simulink model "Initalisation_block"  (R2019b)
settings: Solver=ode3  StartTime=0.0  StopTime=0.01  FixedStep=0.000080  RelTol=1e-3  EnableMultiTasking=on
settings Model: Creator=cary  LastModifiedBy=adshetgaonkar
settings DataIOCC: LimitDataPoints=on  SaveFormat=Array  SignalLoggingSaveFormat=ModelDataLogs  SaveOutput=off  SignalLogging=off  DSMLogging=off  SaveTime=off  ReturnWorkspaceOutputs=off
settings OptimizationCC: ExpressionDepthLimit=2147483647  LifeSpan=1  EfficientTunableParamExpr=on
settings DebuggingCC: UnderspecifiedInitializationDetection=Classic  MergeDetectMultiDrivingBlocksExec=none  SolverPrmCheckMsg=warning  FcnCallInpInsideContextMsg=warning  StateNameClashWarn=warning  SFUnexpectedBacktrackingDiag=warning  SFNoUnconditionalDefaultTransitionDiag=warning  SFExecutionAtInitializationDiag=none  ArithmeticOperatorsInVariantConditions=warning
settings HardwareCC: ProdBitPerPointer=32  ProdBitPerSizeT=32  ProdBitPerPtrDiffT=32  ProdLargestAtomicFloat=None  ProdIntDivRoundTo=Undefined  ProdEndianess=Unspecified  ProdWordSize=32  ProdHWDeviceType=32-bit Generic
settings ModelReferenceCC: PropagateSignalLabelsOutOfModel=off
settings SFSimCC: SimUseLocalCustomCode=off  MATLABDynamicMemAlloc=off  CustomCodeUndefinedFunction=UseInterfaceOnly
settings RTWCC: SystemTargetFile=ert.tlc  TemplateMakefile=ert_default_tmf  RTWUseLocalCustomCode=off
settings CodeAppCC: IgnoreCustomStorageClasses=off  CustomSymbolStrType=$N$R$M  StateflowObjectComments=on  InternalIdentifier=Classic
settings ERTTargetCC: MultiwordLength=2048  GenerateSampleERTMain=on  IncludeMdlTerminateFcn=off  SupportComplex=off  SupportContinuousTime=on  SupportVariableSizeSignals=on  ERTCustomFileTemplate=example_file_process.tlc  ConvertIfToSwitch=off  SuppressUnreachableDefaultCases=off
settings ConfigComp: CovMetricSettings=dw  CovHtmlReporting=on  CovSaveCumulativeToWorkspaceVar=on  CovSaveSingleToWorkspaceVar=on  CovExternalEMLEnable=off

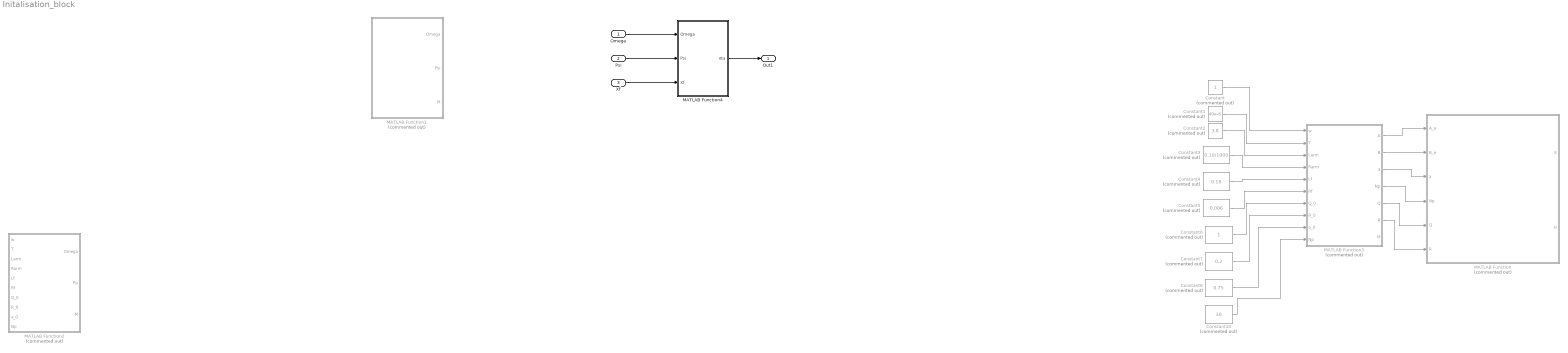
== system Initalisation_block ==
  Omega : Inport  PortDimensions=[20 20]
  Psi : Inport  Port=2  PortDimensions=[20 10]
  Xf : Inport  Port=3  PortDimensions=[10 1]
  Constant : Constant  Commented=on
  Constant1 : Constant  Commented=on  Value=40e-6
  Constant10 : Constant  Commented=on  Value=30
  Constant2 : Constant  Commented=on  Value=3.8
  Constant3 : Constant  Commented=on  Value=0.10/1000
  Constant4 : Constant  Commented=on  Value=0.18
  Constant5 : Constant  Commented=on  Value=0.006
  Constant6 : Constant  Commented=on
  Constant7 : Constant  Commented=on  Value=0.2
  Constant8 : Constant  Commented=on  Value=0.75
  MATLAB Function : MATLAB Function  Commented=on  TreatAsAtomicUnit=on
  MATLAB Function1 : MATLAB Function  Commented=on  TreatAsAtomicUnit=on
  MATLAB Function2 : MATLAB Function  Commented=on  TreatAsAtomicUnit=on
  MATLAB Function3 : MATLAB Function  Commented=on  TreatAsAtomicUnit=on
  MATLAB Function4 : MATLAB Function  TreatAsAtomicUnit=on
  Out1 : Outport  SignalName=eta
  wires:
  MATLAB Function3/1(A) -> MATLAB Function/1(A_e)
  MATLAB Function3/2(B) -> MATLAB Function/2(B_e)
  MATLAB Function3/3(a) -> MATLAB Function/3(a)
  MATLAB Function3/4(Np) -> MATLAB Function/4(Np)
  MATLAB Function3/5(Q) -> MATLAB Function/5(Q)
  MATLAB Function3/6(R) -> MATLAB Function/6(R)
  Constant1/1 -> MATLAB Function3/2(T)
  Constant/1 -> MATLAB Function3/1(w)
  Constant2/1 -> MATLAB Function3/3(Larm)
  Constant3/1 -> MATLAB Function3/4(Rarm)
  Constant4/1 -> MATLAB Function3/5(Lf)
  Constant5/1 -> MATLAB Function3/6(Rf)
  Constant6/1 -> MATLAB Function3/7(Q_0)
  Constant7/1 -> MATLAB Function3/8(R_0)
  Constant8/1 -> MATLAB Function3/9(a_0)
  Constant10/1 -> MATLAB Function3/10("Np ")
  Omega/1 -> MATLAB Function4/1(Omega)
  Psi/1 -> MATLAB Function4/2(Psi)
  Xf/1 -> MATLAB Function4/3(Xf)
  MATLAB Function4/1(eta) -> Out1/1

== matlab function Initalisation_block/MATLAB Function1 ==
  data: Omega output; Psi output; M output [1..100]
function [Omega,Psi,M] = fcn()
D = []; 
D = coder.load('initial_qudratic_papervx.mat');

Omega = D.Omega; 

Psi = D.Psi;

M = D.M;
end

== matlab function Initalisation_block/MATLAB Function2 ==
  data: Omega output; Psi output; w input size=1; M output [1..100]; T input size=1; Larm input size=1; Rarm input size=1; Lf input size=1; Rf input size=1; Q_0 input size=1; R_0 input size=1; a_0 input size=1; Np input size=1
function [Omega,Psi,M] = fcn(w,T,Larm,Rarm,Lf,Rf,Q_0,R_0,a_0,Np)
%w = 1; 
%T =0.2e-3; 
% T = 30e-6; %%%%% very important for simple circuit with 1e-6 it works
% Larm =  1.1;
% Rarm = 0.10/1000

%T = 40e-6; %%%%% very important for simple circuit with 1e-6 it works
%Larm = 3.8;  %%1.5 %%3.8
%Rarm = 0.10/1000; %%%0.10/1000;

%Lf = 0.18;
%Rf = 0.006; %Rf = 0.006;
%%
R_ac_eq = Rf + Rarm/2;  
L_ac_eq = Lf + Larm/2; 
R_dc_eq = 2*Rarm; 
L_dc_eq = 2*Larm;

A_ac = [-Rarm/Larm 2*w 0 0 0; -2*w -Rarm/Larm 0 0 0; 0 0 -Rarm/Larm 0 0; ...
        0 0 0  -R_ac_eq/L_ac_eq -w; 0 0 0 w -R_ac_eq/L_ac_eq ]; 
B_ac = [-1/Larm 0 0 0 0; 0 -1/Larm 0 0 0; 0 0 -1/Larm 0 0;
         0 0 0 1/L_ac_eq 0 ; 0 0 0 0 1/L_ac_eq ];

[Na_r,Na_c] = size(A_ac); 
[Nb_r,Nb_c] = size(B_ac);
C_ac = eye(Na_r,Nb_r); 
D_ac = zeros(Na_r,Nb_c);

F = expm(A_ac*T); 
G = A_ac\((expm(A_ac*T)- eye([Na_r,Na_c]))*B_ac);

Ap_ac = F; 
Bp_ac = G; 
Cp_ac = C_ac; 
%%%%%%%%%%%%%%%%%%%%%%%%%%%%%%%
[m1,n1]=size(Cp_ac);
[n1,n_in]=size(Bp_ac);
A=eye(n1+m1,n1+m1);
A(1:n1,1:n1)=Ap_ac;
A(n1+1:n1+m1,1:n1)=Cp_ac*Ap_ac;
B=zeros(n1+m1,n_in);
B(1:n1,:)=Bp_ac;
B(n1+1:n1+m1,:)=Cp_ac*Bp_ac;
C=zeros(m1,n1+m1);
C(:,n1+1:n1+m1)=eye(m1,m1);

%%
%Q_0 = 1;
%R_0 = 0.2;
%a_0 =0.75;
Q= Q_0*C'*C;
%Q=[0 0 0 0; 0 0 0 0; 0 0 100 0;  0 0 0 100]; %% check for effect of Q 
R=R_0*eye(n_in,n_in);
%R=0.9*eye(n_in,n_in)
a=a_0*ones (n_in,1);
N= 4*ones (n_in,1); %you can increase N
%Np=45;
%Np=30;
[Omega,Psi]= dmpc(A,B,a,N,Np,Q,R); 
%%%
%%
xm=zeros(n1,1);
N_sim = 300;
y=zeros(m1,1);
u=zeros(n_in,1);
xm=zeros(n1,1);
%%%%%%%%%%refrence %%%%%%%

r = zeros(m1,1);
Xf=[xm;(y-r)];
u_min= -0.3*ones (n_in,1);
u_max= 0.3*ones (n_in,1);
deltau_min = -10*ones (n_in,1);
deltau_max = 10*ones (n_in,1);
up=zeros(n_in,1);
%[M,Lzerot]=Mdu(a,N,n_in,1); %% for contrain on the rate
%[M0]= Mu(a,N,n_in,2); %%% for contrain on the amplitude 
%% contrain on both rate and amplitude
[M1,Lzerot]=Mdu(a,N,n_in,1);
M0=Mu(a,N,n_in,1);
M=[M0;-M0;M1;-M1];

end

== matlab function Initalisation_block/MATLAB Function ==
  data: A_e input; E output; B_e input; a input; Np input; Q input; R input; H output
 function [E,H] =fcn(A_e,B_e,a,Np,Q,R)
%A_e;B_e define the extended state-space model when
% integrator is used
%they can also be other forms of state-space models
% a contains the Laguerre pole locations for each input
%N the number of terms for each input
%Np prediction horizon
%Q weight on the state variables
%R weight on the input variables assumed to be diagonal.
% The cost function is J= eta ^T E eta +2 eta ^T H x(k_i)
[n,n_in]=size(B_e);
N= 4*ones (n_in,1);
N_pa=sum(N); %the dimension of eta
E=zeros(N_pa,N_pa);
H=zeros(N_pa,n);
R_para=zeros(N_pa,N_pa);
n0=1;
ne=N(1);
for i=1:n_in-1
R_para(n0:ne,n0:ne)= R(i,i)*eye(N(i),N(i));
n0=n0+N(i);
ne=ne+N(i+1);
end
R_para(n0:N_pa,n0:N_pa)=R(n_in,n_in)*eye(N(n_in),N(n_in));
S_in=zeros(n,N_pa);
[Al,L0]=lagd(a(1),N(1));
S_in(:,1:N(1))=B_e(:,1)*L0';
In_s=1;
for jj=2:n_in
[Al,L0]=lagd(a(jj),N(jj));
In_s=N(jj-1)+In_s;
In_e=In_s+N(jj)-1;
S_in(:,In_s:In_e)=B_e(:,jj)*L0';
end
S_sum = S_in;
phi=S_in;
E=(phi)'*Q*(phi);
H=phi'*Q*A_e;
for i=2:Np
Eae=A_e^i;
%calculate the finite sum S for each input
%%%%%%%%%%%%%%%%%%%%%%%%%%%%%%%%%%%%%%%
%For each sample i
%%%%%%%%%%%%calculate input number 1
%specify the L0 and state matrix Al
%associated with the first input
[Al,L0]=lagd(a(1),N(1));
% Laguerre function associated with input number 1
S_sum(:,1:N(1))=A_e*S_sum(:,1:N(1))+ S_in(:,1:N(1))*(Al^(i-1))';
%%move on to input number 2 and so on
In_s=1;
for kk=2:n_in
[Al,L0]=lagd(a(kk),N(kk));
In_s=N(kk-1)+In_s;
In_e=In_s+N(kk)-1;
S_sum(:,In_s:In_e)=A_e*S_sum(:,In_s:In_e)+ S_in(:,In_s:In_e)*(Al^(i-1))';
end
phi=S_sum;
E=E+phi'*Q*phi;
H=H+phi'*Q*Eae;
end
E=E+R_para;

== matlab function Initalisation_block/MATLAB Function3 ==
  data: w input; A output; T input; Larm input; Rarm input; Lf input; Rf input; Q_0 input; R_0 input; a_0 input; B output; a output; Np output; Q output; R output; Np input; M output
function [A,B,a,Np,Q,R,M] = fcn(w,T,Larm,Rarm,Lf,Rf,Q_0,R_0,a_0,Np)
%w = 1; 
%T =0.2e-3; 
% T = 30e-6; %%%%% very important for simple circuit with 1e-6 it works
% Larm =  1.1;
% Rarm = 0.10/1000

%T = 40e-6; %%%%% very important for simple circuit with 1e-6 it works
%Larm = 3.8;  %%1.5 %%3.8
%Rarm = 0.10/1000; %%%0.10/1000;

%Lf = 0.18;
%Rf = 0.006; %Rf = 0.006;
%%
R_ac_eq = Rf + Rarm/2;  
L_ac_eq = Lf + Larm/2; 
R_dc_eq = 2*Rarm; 
L_dc_eq = 2*Larm;

A_ac = [-Rarm/Larm 2*w 0 0 0; -2*w -Rarm/Larm 0 0 0; 0 0 -Rarm/Larm 0 0; ...
        0 0 0  -R_ac_eq/L_ac_eq -w; 0 0 0 w -R_ac_eq/L_ac_eq ]; 
B_ac = [-1/Larm 0 0 0 0; 0 -1/Larm 0 0 0; 0 0 -1/Larm 0 0;
         0 0 0 1/L_ac_eq 0 ; 0 0 0 0 1/L_ac_eq ];

[Na_r,Na_c] = size(A_ac); 
[Nb_r,Nb_c] = size(B_ac);
C_ac = eye(Na_r,Nb_r); 
D_ac = zeros(Na_r,Nb_c);

F = expm(A_ac*T); 
G = A_ac\((expm(A_ac*T)- eye([Na_r,Na_c]))*B_ac);

Ap_ac = F; 
Bp_ac = G; 
Cp_ac = C_ac; 
%%%%%%%%%%%%%%%%%%%%%%%%%%%%%%%
[m1,n1]=size(Cp_ac);
[n1,n_in]=size(Bp_ac);
A=eye(n1+m1,n1+m1);
A(1:n1,1:n1)=Ap_ac;
A(n1+1:n1+m1,1:n1)=Cp_ac*Ap_ac;
B=zeros(n1+m1,n_in);
B(1:n1,:)=Bp_ac;
B(n1+1:n1+m1,:)=Cp_ac*Bp_ac;
C=zeros(m1,n1+m1);
C(:,n1+1:n1+m1)=eye(m1,m1);

%%
%Q_0 = 1;
%R_0 = 0.2;
%a_0 =0.75;
Q= Q_0*C'*C;
%Q=[0 0 0 0; 0 0 0 0; 0 0 100 0;  0 0 0 100]; %% check for effect of Q 
R=R_0*eye(n_in,n_in);
%R=0.9*eye(n_in,n_in)
a=a_0*ones (n_in,1);

xm=zeros(n1,1);
N_sim = 300;
y=zeros(m1,1);
u=zeros(n_in,1);
xm=zeros(n1,1);
%%%%%%%%%%refrence %%%%%%%

r = zeros(m1,1)
Xf=[xm;(y-r)]
u_min= -0.3*ones (n_in,1);
u_max= 0.3*ones (n_in,1);
deltau_min = -10*ones (n_in,1);
deltau_max = 10*ones (n_in,1);
up=zeros(n_in,1);
%[M,Lzerot]=Mdu(a,N,n_in,1); %% for contrain on the rate
%[M0]= Mu(a,N,n_in,2); %%% for contrain on the amplitude 
%% contrain on both rate and amplitude
N=4*ones (n_in,1);
[M1,Lzerot]= Mdu(a,N,n_in,1);
M0=Mu(a,N,n_in,1);
M=[M0;-M0;M1;-M1];

== matlab function Initalisation_block/MATLAB Function4 ==
  data: Omega input; eta output; Psi input; Xf input
function eta  = fcn(Omega,Psi,Xf)
eta= -(Omega\Psi)*(Xf);
end
